simulink model "trail1"  (R2023a)
settings: Solver=FixedStepAuto  StartTime=0.0  StopTime=10.0  RelTol=1e-3
undefined symbols (not defined in the file): Data_Display, Data_Display1, Data_Display2, untitled
libraries: androidsensorlib x4, androiduilib x3, dspfdesign x2
settings Model: Creator=Shesh  LastModifiedBy=Shesh
settings OptimizationCC: EnhancedBackFolding=on  PassReuseOutputArgsAs=Individual arguments  ZeroExternalMemoryAtStartup=off  ZeroInternalMemoryAtStartup=off  MaxStackSize=64  OptimizeBlockOrder=speed  DifferentSizesBufferReuse=on  OptimizationCustomize=off  EfficientTunableParamExpr=on
settings DebuggingCC: ParameterTunabilityLossMsg=error
settings HardwareCC: ProdBitPerPointer=32  ProdBitPerSizeT=32  ProdBitPerPtrDiffT=32  ProdLargestAtomicInteger=Long  ProdLargestAtomicFloat=Double  ProdWordSize=32  ProdHWDeviceType=ARM Compatible->ARM Cortex
settings SFSimCC: MATLABDynamicMemAlloc=off
settings RTWCC: Description=Embedded Coder  SystemTargetFile=ert.tlc  HardwareBoard=Android Device  TLCOptions="-aInlineSetEventsForThisBaseRateFcn=TLC_FALSE -aSuppressMultiTaskScheduler=TLC_FALSE  -aRateBasedStepFcn=0"  TemplateMakefile=ert_default_tmf  RTWVerbose=off  Toolchain=Android SDK/NDK Tools
settings CodeAppCC: ForceParamTrailComments=on  IgnoreCustomStorageClasses=off  OperatorAnnotations=on  SimulinkDataObjDesc=on  SFDataObjDesc=on  InsertBlockDesc=on

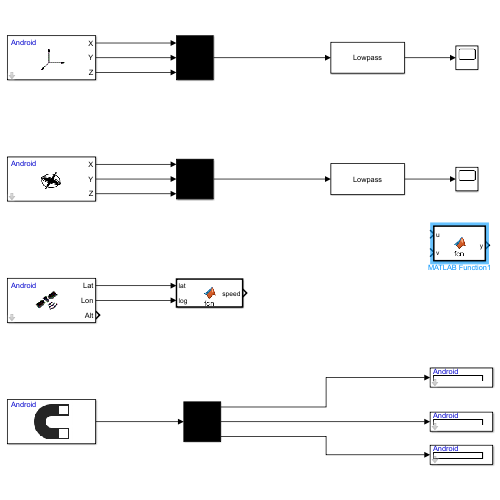
[thumbnail: Simulink's stored preview of the top-level diagram]
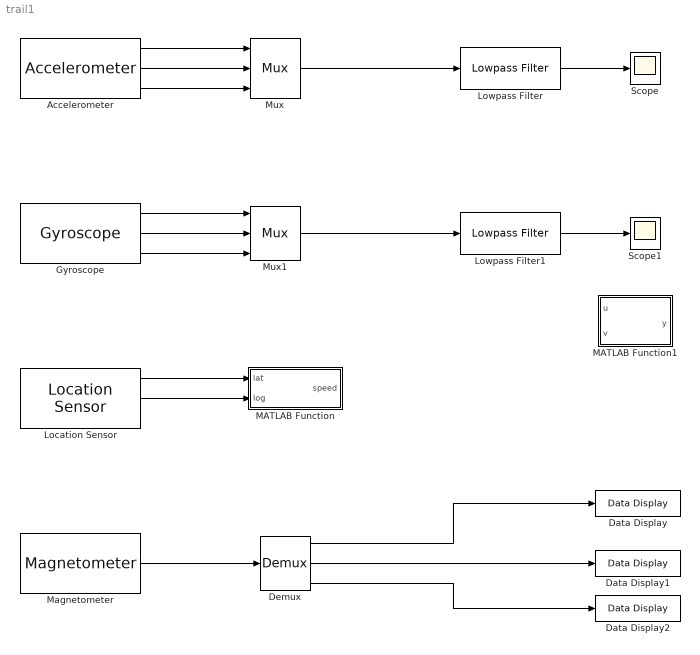
== system trail1 ==
  Accelerometer : androidsensorlib/Accelerometer  OutputVector=off  SampleTime=0.01  BlockPlatform=Android
  Data Display : androiduilib/Data Display  DataDisplayId=untitled/Data_Display  Format=Float  Precision=6  SimulateUsing=Code generation  blockPlatform=Android
  Data Display1 : androiduilib/Data Display  DataDisplayId=untitled/Data_Display1  Format=Float  Precision=6  SimulateUsing=Code generation  blockPlatform=Android
  Data Display2 : androiduilib/Data Display  DataDisplayId=untitled/Data_Display2  Format=Float  Precision=6  SimulateUsing=Code generation  blockPlatform=Android
  Demux : Demux  Outputs=3
  Gyroscope : androidsensorlib/Gyroscope  OutputVector=off  SampleTime=0.01  BlockPlatform=Android
  Location Sensor : androidsensorlib/Location Sensor  OutputVector=off  SampleTime=0.01  BlockPlatform=Android
  Lowpass Filter : dspfdesign/Lowpass Filter  FilterType=FIR  DesignForMinimumOrder=on  FilterOrder=50  PassbandFrequency=8e3  StopbandFrequency=12e3  PassbandRipple=0.1  StopbandAttenuation=80  SampleRateMode=Specify on dialog  SampleRate=44100  SimulateUsing=Interpreted execution  roundingMode=Floor  coeffsDataTypeStr=fixdt(1,16)
  Lowpass Filter1 : dspfdesign/Lowpass Filter  FilterType=FIR  DesignForMinimumOrder=on  FilterOrder=50  PassbandFrequency=8e3  StopbandFrequency=12e3  PassbandRipple=0.1  StopbandAttenuation=80  SampleRateMode=Specify on dialog  SampleRate=44100  SimulateUsing=Interpreted execution  roundingMode=Floor  coeffsDataTypeStr=fixdt(1,16)
  MATLAB Function : MATLAB Function  TreatAsAtomicUnit=on
  MATLAB Function1 : MATLAB Function  TreatAsAtomicUnit=on
  Magnetometer : androidsensorlib/Magnetometer  SampleTime=0.01
  Mux : Mux  Inputs=3
  Mux1 : Mux  Inputs=3
  Scope : Scope
  Scope1 : Scope
  wires:
  Accelerometer/1 -> Mux/1
  Accelerometer/2 -> Mux/2
  Accelerometer/3 -> Mux/3
  Gyroscope/1 -> Mux1/1
  Gyroscope/2 -> Mux1/2
  Gyroscope/3 -> Mux1/3
  Mux/1 -> Lowpass Filter/1
  Mux1/1 -> Lowpass Filter1/1
  Location Sensor/1 -> MATLAB Function/1(lat)
  Location Sensor/2 -> MATLAB Function/2(log)
  Magnetometer/1 -> Demux/1
  Demux/1 -> Data Display/1
  Demux/2 -> Data Display1/1
  Demux/3 -> Data Display2/1
  Lowpass Filter1/1 -> Scope1/1
  Lowpass Filter/1 -> Scope/1

== matlab function trail1/MATLAB Function ==
  data: lat input; speed output; log input
function speed = fcn(lat, log)

speed = lat+log;

== matlab function trail1/MATLAB Function1 ==
  data: u input; y output; v input
function y = fcn(u, v)

y = 1;
